simulink model "autopilot_2"  (R2019a)
settings: Solver=VariableStepAuto  StartTime=0.0  StopTime=300  RelTol=1e-3
values from neighbouring files (symbols this model uses):
  C = [ ... (first row only)    [Problem_2.m]    (also in gen_measurement.m = [0 0 1 0; init_kalman.m = [0 0 1 0; kalman_K.m = [0 0 1 0; matrices.mat = [0  0  1  0; 0  0  0  1])
  chi_c = deg2rad(10)    [Problem_2.m]
  d = deg2rad(1.5)    [Problem_2.m]
  DELTA = [    0.0000 ... (first row only)    [kalman_K.m]    (also in matrices.mat = [2.01719397305e-05 -3.21953461389e-05 -0.0064091191103 -0.00)
  g = 9.81    [Problem_2.m]
  GAMMA = [1 0 0 0 0 1 0 0 0 0 1 0 ... (16 elements, 4x4)]    [matrices.mat]
  initial_P = initial_state * initial_state'    [init_kalman.m]
  initial_state = [0,0,0,0]'    [init_kalman.m]
  k_d_phi = 1.9351    [Problem_2.m]
  k_i_chi = (w_n_chi^2*V_g)/g    (= 0.21351016627)    [Problem_2.m]
  k_p_chi = (2*zeta_chi*w_n_chi*V_g)/g    (= 3.74513534942)    [Problem_2.m]
  k_p_phi = -2    [Problem_2.m]
  PHI = [0.9964    0.0005    0.0003   -0.0112 ... (first row only)    [kalman_K.m]    (also in matrices.mat = [0.996386897181 -0.000524187110195 -0.104154311891 0.0684916)
  Q = Ts*10^-6*mat    [init_kalman.m]
  R = 0.2^2*eye(2)    [gen_measurement.m]    (also in init_kalman.m)
  V_g = 580/3.6    (= 161.111111111)    [Problem_2.m]
libraries: simulink x1
settings Model: Creator=joaki  LastModifiedBy=magnusknaedal

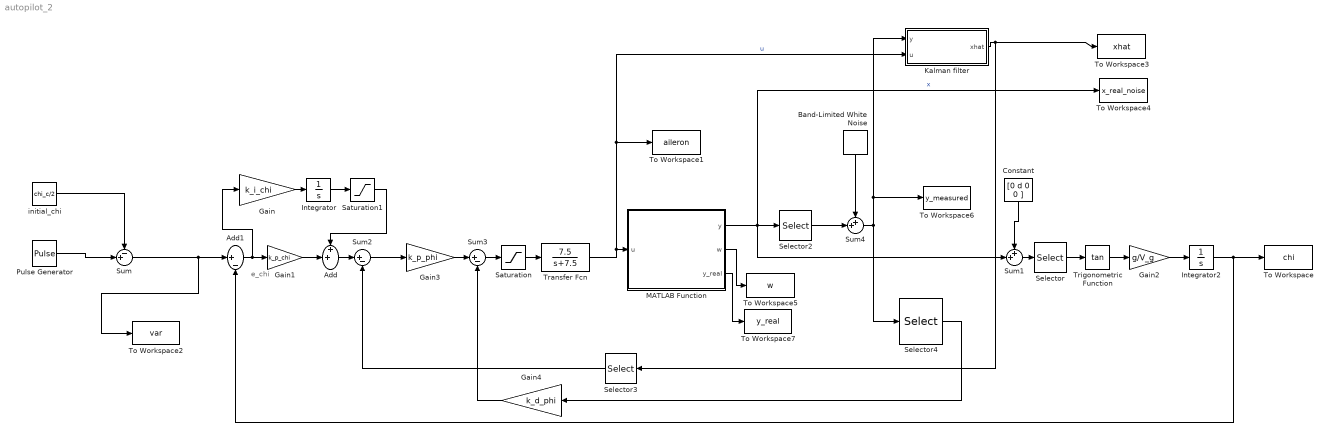
== system autopilot_2 ==
  note: e_chi
  Add : Sum  Inputs=++|
  Add1 : Sum  Inputs=|+-
  Band-Limited White Noise : simulink/Sources/Band-Limited White Noise  Cov=[0.0035]  Ts=0.01  seed=[23341]
  Constant : Constant  Value=[0 d 0 0 ]
  Gain : Gain  Gain=k_i_chi
  Gain1 : Gain  Gain=k_p_chi
  Gain2 : Gain  Gain=g/V_g
  Gain3 : Gain  Gain=k_p_phi
  Gain4 : Gain  Gain=k_d_phi
  Integrator : Integrator
  Integrator2 : Integrator
  Kalman filter : Subsystem
  MATLAB Function : MATLAB Function  TreatAsAtomicUnit=on
  Pulse Generator : DiscretePulseGenerator  PulseType=Time based  Amplitude=chi_c  Period=200  PulseWidth=50
  Saturation : Saturate  UpperLimit=30*pi/180  LowerLimit=-30*pi/180
  Saturation1 : Saturate  UpperLimit=inf  LowerLimit=-inf
  Selector : Selector  InputPortWidth=4  IndexOptions=Index vector (dialog)  Indices=[2]  OutputSizes=1
  Selector2 : Selector  InputPortWidth=4  IndexOptions=Index vector (dialog)  Indices=[3 4]  OutputSizes=1
  Selector3 : Selector  InputPortWidth=4  IndexOptions=Index vector (dialog)  Indices=[2]  OutputSizes=1
  Selector4 : Selector  InputPortWidth=2  IndexOptions=Index vector (dialog)  Indices=[1]  OutputSizes=1
  Sum : Sum  Inputs=-+|
  Sum1 : Sum  Inputs=++|
  Sum2 : Sum  Inputs=|+-
  Sum3 : Sum  Inputs=|+-
  Sum4 : Sum  Inputs=++|
  To Workspace : ToWorkspace  VariableName=chi  SaveFormat=Timeseries  SampleTime=-1
  To Workspace1 : ToWorkspace  VariableName=aileron  SaveFormat=Timeseries  SampleTime=-1
  To Workspace2 : ToWorkspace  VariableName=var  SaveFormat=Structure With Time  SampleTime=-1
  To Workspace3 : ToWorkspace  VariableName=xhat  SaveFormat=Timeseries  SampleTime=-1
  To Workspace4 : ToWorkspace  VariableName=x_real_noise  SaveFormat=Timeseries  SampleTime=-1
  To Workspace5 : ToWorkspace  VariableName=w  SaveFormat=Timeseries  SampleTime=-1
  To Workspace6 : ToWorkspace  VariableName=y_measured  SaveFormat=Timeseries  SampleTime=-1
  To Workspace7 : ToWorkspace  VariableName=y_real  SaveFormat=Timeseries  SampleTime=-1
  Transfer Fcn : TransferFcn  Numerator=[7.5]  Denominator=[1 7.5]
  Trigonometric Function : Trigonometry  Operator=tan
  "initial_chi " : Constant  Value=chi_c/2
  wires:
  Gain/1 -> Integrator/1
  Add1/1 -> Gain/1, Gain1/1
  Integrator2/1 -> To Workspace/1, Add1/2
  Gain2/1 -> Integrator2/1
  Trigonometric Function/1 -> Gain2/1
  Saturation/1 -> Transfer Fcn/1
  Selector/1 -> Trigonometric Function/1
  Sum1/1 -> Selector/1
  Pulse Generator/1 -> Sum/2
  "initial_chi "/1 -> Sum/1
  Sum/1 -> Add1/1, To Workspace2/1
  Transfer Fcn/1 -> Kalman filter/2(u), To Workspace1/1, MATLAB Function/1(u)  "u"
  Integrator/1 -> Saturation1/1
  Saturation1/1 -> Add/1
  Sum2/1 -> Gain3/1
  Sum3/1 -> Saturation/1
  MATLAB Function/1(y) -> To Workspace4/1, Sum1/2, Selector2/1  "x"
  Selector4/1 -> Gain4/1
  Gain4/1 -> Sum3/2
  Gain1/1 -> Add/2
  Add/1 -> Sum2/1
  Gain3/1 -> Sum3/1
  Selector2/1 -> Sum4/2
  Band-Limited White Noise/1 -> Sum4/1
  Sum4/1 -> Selector4/1, To Workspace6/1, Kalman filter/1(y)
  MATLAB Function/2(w) -> To Workspace5/1
  MATLAB Function/3(y_real) -> To Workspace7/1
  Selector3/1 -> Sum2/2
  Kalman filter/1(xhat) -> To Workspace3/1, Selector3/1
  Constant/1 -> Sum1/1

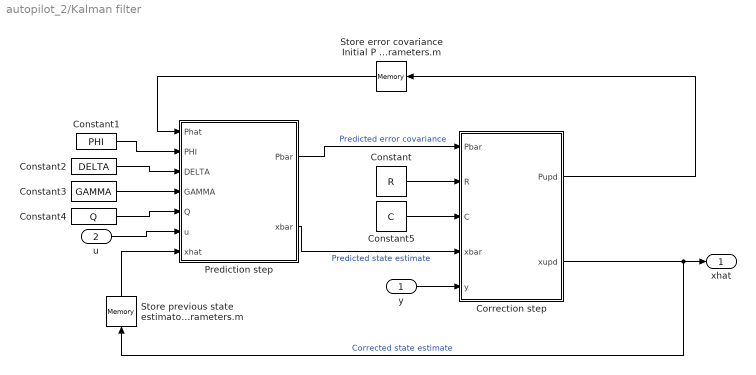
== system autopilot_2/Kalman filter ==
  y : Inport
  u : Inport  Port=2
  Constant : Constant  Value=R
  Constant1 : Constant  Value=PHI
  Constant2 : Constant  Value=DELTA
  Constant3 : Constant  Value=GAMMA
  Constant4 : Constant  Value=Q
  Constant5 : Constant  Value=C
  Correction step : MATLAB Function  TreatAsAtomicUnit=on
  Prediction step : MATLAB Function  TreatAsAtomicUnit=on
  Store error covariance Initial P set in parameters.m : Memory  InitialCondition=initial_P
  Store previous state estimaton Initial state set in parameters.m : Memory  InitialCondition=initial_state
  xhat : Outport
  wires:
  u/1 -> Prediction step/6(u)
  Store previous state estimaton Initial state set in parameters.m/1 -> Prediction step/7(xhat)
  Prediction step/2(xbar) -> Correction step/4(xbar)  "Predicted state estimate"
  Prediction step/1(Pbar) -> Correction step/1(Pbar)  "Predicted error covariance"
  Correction step/1(Pupd) -> Store error covariance Initial P set in parameters.m/1
  y/1 -> Correction step/5(y)
  Correction step/2(xupd) -> Store previous state estimaton Initial state set in parameters.m/1, xhat/1  "Corrected state estimate"
  Store error covariance Initial P set in parameters.m/1 -> Prediction step/1(Phat)
  Constant/1 -> Correction step/2(R)
  Constant1/1 -> Prediction step/2(PHI)
  Constant2/1 -> Prediction step/3(DELTA)
  Constant3/1 -> Prediction step/4(GAMMA)
  Constant4/1 -> Prediction step/5(Q)
  Constant5/1 -> Correction step/3(C)

== matlab function autopilot_2/Kalman filter/Correction step ==
  data: Pbar input; R input; C input; xbar input; Pupd output; y input; xupd output
function [Pupd, xupd] = update(Pbar,R, C,xbar,y)
% returns the mean and covariance after correcting based on the
% measurement, ref Fossen 2011 table 11.1

K = (Pbar * C')/(C * Pbar * C' + R);
xupd = xbar + K * (y - C * xbar);

I = eye(size(Pbar));
Pupd = (I - K * C) * Pbar * (I - K * C)' + K*R*K';

end

== matlab function autopilot_2/MATLAB Function ==
  settings: updateMethod=DISCRETE
  data: u input; y output; w output; y_real output
function [y, w, y_real] = state_space(u)
% Generate the output of the state space

    % Persistent variables to be kept between function calls
    persistent counter; % Variable for checking if it is the first iteration.
    persistent x;       % The state x
    persistent x_real;
    
   % The next line is necessary for generating unique process noise for every simulation.
   % Otherwise, the noise will be equal every time you run the simulation,
   % even though it is white. This has to do with how Matlab generates
   % random numbers. 
   coder.extrinsic('randn','rng');
    
    h = 0.01;       % Time step of Euler integration
    delta_a_c = u;  % Aileron input
    Ed = eye(5);
    if isempty(counter)
      % First iteration
        counter = 1;
           
        % Initialize state space
        x = zeros(5,1);
        w = zeros(5,1); 
        x_real = zeros(5,1);
        rng('shuffle'); % Necessary for generating unique process noise for every simulation.
    else
        % State-space matrices
        A = [-0.322, 0.052, 0.028, -1.12, 0.002;
             0, 0, 1, -0.001, 0;
             -10.6, 0, -2.87, 0.46, -0.65;
             6.87, 0, -0.04, -0.32, -0.02;
             0, 0, 0, 0, -7.5];
 
        B = [0; 0; 0; 0; 7.5;];
        
        E = eye(5);
        
        % Discrete version
        Ad = eye(5) + h*A;
        Bd = h*B;
        Ed = E;
        
        % The Qd matrix in the assignment is given directly in discrete-time here and
        % therefore, it is not necessary to discretize E.
        Qd = h*10^-6*[0.001, 0, 0, 0, 0;
                  0, 1, 0, 0, 0;
                  0, 0, 100, 0, 0;
                  0, 0, 0, 10, 0;
                  0, 0, 0, 0, 0];
          
        w = sqrt(Qd)*randn(5,1,1); % The standard deviation must be multiplied with random numbers with a zero-mean unit variance random number to generate process noise. 
        
        % Discrete-time state space update
        x_real = Ad*x_real + Bd * delta_a_c;
        x = Ad*x + Bd * delta_a_c + Ed*w;
        
    end
    y = x(1:4); % Return every state except the actuator state.
    
    y_real = x_real(1:4);
    %w = w;
    
end

== matlab function autopilot_2/Kalman filter/Prediction step ==
  data: Pbar output; Phat input; PHI input; DELTA input; GAMMA input; Q input; u input; xhat input; xbar output
function [Pbar, xbar] = predict(Phat,PHI,DELTA,GAMMA,Q,u, xhat)
% returns the predicted mean (=state) and covariance (-covariance of 
% predicted state estimate error) for a time step Ts, ref Fossen 2011 table 11.1

% PREDICTION
xbar = PHI * xhat + DELTA * u;
Pbar = PHI * Phat * PHI' + GAMMA * Q * GAMMA';

end
